simulink model "Observer"  (R2016b)
settings: Solver=VariableStepAuto  StartTime=0.0  StopTime=10.0  RelTol=1e-3
undefined symbols (not defined in the file or in its folder): A_c, A_d, B_c, B_d, C_c, C_d, D_c, L, Ts
settings Model: Creator=Ashraf  LastModifiedBy=Ashraf

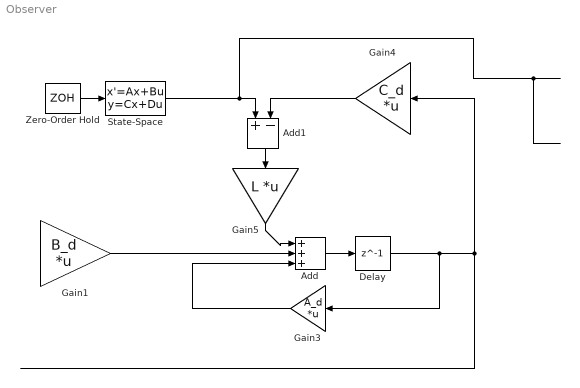
== system Observer ==
  Add : Sum  Inputs=+++
  Add1 : Sum  Inputs=+-
  Delay : Delay  DelayLength=1  SampleTime=Ts
  Gain1 : Gain  Gain=B_d  Multiplication=Matrix(K*u)
  Gain3 : Gain  Gain=A_d  Multiplication=Matrix(K*u)
  Gain4 : Gain  Gain=C_d  Multiplication=Matrix(K*u)
  Gain5 : Gain  Gain=L  Multiplication=Matrix(K*u)
  State-Space : StateSpace  A=A_c  B=B_c  C=C_c  D=D_c  X0=0
  Zero-Order Hold : ZeroOrderHold  SampleTime=-1
  wires:
  Delay/1 -> Gain4/1, Gain3/1
  Add/1 -> Delay/1
  Gain4/1 -> Add1/2
  Add1/1 -> Gain5/1
  Gain5/1 -> Add/1
  Gain1/1 -> Add/2
  Gain3/1 -> Add/3
  State-Space/1 -> Add1/1
  Zero-Order Hold/1 -> State-Space/1
  ? -> Zero-Order Hold/1, Gain1/1
